simulink model "ieee80211n"  (Simulink 6.0)
settings: Solver=VariableStepDiscrete  StartTime=0.0  StopTime=inf  RelTol=1e-3
PreLoadFcn:
  | load IEEE80211n_init;
values from neighbouring files (symbols this model uses):
  params =     [IEEE80211n_init.mat]    (also in IEEE80211n_settings.m = p)
undefined symbols (not defined in the file or in its folder): magnitude
libraries: commblkintrlv2 x196, dspsigops x143, simulink x136, commdigbbndam2 x98, dspmtrx3 x96, dspsigattribs x69, dspstat3 x38, commutil2 x32, commsequence2 x26, commcnvcod2 x10, dspindex x9, dspmlti3 x8
(part 9 of 12)

== system ieee80211n/MIMODetection/Channel Estimation/ChannelEst10 ==
  trainsig : Inport  Port=1  LatchInput=off
  rxsig : Inport  Port=2  LatchInput=off
  Channel estimates : Subsystem
  Product1 : Product  Inputs=**  SaturateOnIntegerOverflow=on
  Remove DC component : Selector  InputType=Matrix  Elements=[1:26 27:]  Rows=[1:28 30:57]  Columns=-1  InputPortWidth=53
  Remove training DC component : Selector  InputType=Matrix  Elements=[1:26 27:]  Rows=[1:28 30:57]  Columns=-1  InputPortWidth=53
  Select training/data : S-Function  AncestorBlock=dspindex/Multiport Selector  FunctionName=sdspmultiportsel  Parameters=rowsOrCols, numOutports, flatIdxVect, flatLenVect, idxErrMode  mask(Multiport Selector){rowsOrCols=Columns, idxCellArray={params.OFDM_TotPreamblePerFrame-params.OFDM_HTLTF_SymPerFrame+1:params.OFDM_TotPreamblePerFrame}, idxErrMode=Clip Index}
      mask prompts: rowsOrCols "Select:"; idxCellArray "Indices to output:"; idxErrMode "Invalid index:"
      mask help: Output specified rows or columns to one or more output ports. The number of output ports is determined by the number of index vectors, each specified as a separate vector entry in a cell array. Indices are 1-based and need not be unique.
      mask init:
      | [numOutports, flatLenVect, flatIdxVect] = dspblkmultiportsel(idxCellArray);
      mask Help: web(dspbhelp);
      mask StyleString: popup(Rows|Columns),edit,popup(Clip Index|Clip and Warn|Generate Error)
      mask Display: disp(['Select\n' &1]);
  out : Outport
  wires:
  rxsig/1 -> Remove DC component/1
  Channel estimates/1(ch est) -> out/1
  trainsig/1 -> Remove training DC component/1
  Product1/1 -> Channel estimates/2(in)
  Select training/data/1 -> Product1/2
  Remove DC component/1 -> Select training/data/1
  Remove training DC component/1 -> Product1/1, Channel estimates/1(trn)

== system ieee80211n/MIMODetection/Channel Estimation/ChannelEst11 ==
  trainsig : Inport  Port=1  LatchInput=off
  rxsig : Inport  Port=2  LatchInput=off
  Channel estimates : Subsystem
  Product1 : Product  Inputs=**  SaturateOnIntegerOverflow=on
  Remove DC component : Selector  InputType=Matrix  Elements=[1:26 27:]  Rows=[1:28 30:57]  Columns=-1  InputPortWidth=53
  Remove training DC component : Selector  InputType=Matrix  Elements=[1:26 27:]  Rows=[1:28 30:57]  Columns=-1  InputPortWidth=53
  Select training/data : S-Function  AncestorBlock=dspindex/Multiport Selector  FunctionName=sdspmultiportsel  Parameters=rowsOrCols, numOutports, flatIdxVect, flatLenVect, idxErrMode  mask(Multiport Selector){rowsOrCols=Columns, idxCellArray={params.OFDM_TotPreamblePerFrame-params.OFDM_HTLTF_SymPerFrame+1:params.OFDM_TotPreamblePerFrame}, idxErrMode=Clip Index}
      mask prompts: rowsOrCols "Select:"; idxCellArray "Indices to output:"; idxErrMode "Invalid index:"
      mask help: Output specified rows or columns to one or more output ports. The number of output ports is determined by the number of index vectors, each specified as a separate vector entry in a cell array. Indices are 1-based and need not be unique.
      mask init:
      | [numOutports, flatLenVect, flatIdxVect] = dspblkmultiportsel(idxCellArray);
      mask Help: web(dspbhelp);
      mask StyleString: popup(Rows|Columns),edit,popup(Clip Index|Clip and Warn|Generate Error)
      mask Display: disp(['Select\n' &1]);
  out : Outport
  wires:
  rxsig/1 -> Remove DC component/1
  Channel estimates/1(ch est) -> out/1
  trainsig/1 -> Remove training DC component/1
  Product1/1 -> Channel estimates/2(in)
  Select training/data/1 -> Product1/2
  Remove DC component/1 -> Select training/data/1
  Remove training DC component/1 -> Product1/1, Channel estimates/1(trn)

== system ieee80211n/MIMODetection/Channel Estimation/ChannelEst12 ==
  trainsig : Inport  Port=1  LatchInput=off
  rxsig : Inport  Port=2  LatchInput=off
  Channel estimates : Subsystem
  Product1 : Product  Inputs=**  SaturateOnIntegerOverflow=on
  Remove DC component : Selector  InputType=Matrix  Elements=[1:26 27:]  Rows=[1:28 30:57]  Columns=-1  InputPortWidth=53
  Remove training DC component : Selector  InputType=Matrix  Elements=[1:26 27:]  Rows=[1:28 30:57]  Columns=-1  InputPortWidth=53
  Select training/data : S-Function  AncestorBlock=dspindex/Multiport Selector  FunctionName=sdspmultiportsel  Parameters=rowsOrCols, numOutports, flatIdxVect, flatLenVect, idxErrMode  mask(Multiport Selector){rowsOrCols=Columns, idxCellArray={params.OFDM_TotPreamblePerFrame-params.OFDM_HTLTF_SymPerFrame+1:params.OFDM_TotPreamblePerFrame}, idxErrMode=Clip Index}
      mask prompts: rowsOrCols "Select:"; idxCellArray "Indices to output:"; idxErrMode "Invalid index:"
      mask help: Output specified rows or columns to one or more output ports. The number of output ports is determined by the number of index vectors, each specified as a separate vector entry in a cell array. Indices are 1-based and need not be unique.
      mask init:
      | [numOutports, flatLenVect, flatIdxVect] = dspblkmultiportsel(idxCellArray);
      mask Help: web(dspbhelp);
      mask StyleString: popup(Rows|Columns),edit,popup(Clip Index|Clip and Warn|Generate Error)
      mask Display: disp(['Select\n' &1]);
  out : Outport
  wires:
  rxsig/1 -> Remove DC component/1
  Channel estimates/1(ch est) -> out/1
  trainsig/1 -> Remove training DC component/1
  Product1/1 -> Channel estimates/2(in)
  Select training/data/1 -> Product1/2
  Remove DC component/1 -> Select training/data/1
  Remove training DC component/1 -> Product1/1, Channel estimates/1(trn)

== system ieee80211n/MIMODetection/Channel Estimation/ChannelEst13 ==
  trainsig : Inport  Port=1  LatchInput=off
  rxsig : Inport  Port=2  LatchInput=off
  Channel estimates : Subsystem
  Product1 : Product  Inputs=**  SaturateOnIntegerOverflow=on
  Remove DC component : Selector  InputType=Matrix  Elements=[1:26 27:]  Rows=[1:28 30:57]  Columns=-1  InputPortWidth=53
  Remove training DC component : Selector  InputType=Matrix  Elements=[1:26 27:]  Rows=[1:28 30:57]  Columns=-1  InputPortWidth=53
  Select training/data : S-Function  AncestorBlock=dspindex/Multiport Selector  FunctionName=sdspmultiportsel  Parameters=rowsOrCols, numOutports, flatIdxVect, flatLenVect, idxErrMode  mask(Multiport Selector){rowsOrCols=Columns, idxCellArray={params.OFDM_TotPreamblePerFrame-params.OFDM_HTLTF_SymPerFrame+1:params.OFDM_TotPreamblePerFrame}, idxErrMode=Clip Index}
      mask prompts: rowsOrCols "Select:"; idxCellArray "Indices to output:"; idxErrMode "Invalid index:"
      mask help: Output specified rows or columns to one or more output ports. The number of output ports is determined by the number of index vectors, each specified as a separate vector entry in a cell array. Indices are 1-based and need not be unique.
      mask init:
      | [numOutports, flatLenVect, flatIdxVect] = dspblkmultiportsel(idxCellArray);
      mask Help: web(dspbhelp);
      mask StyleString: popup(Rows|Columns),edit,popup(Clip Index|Clip and Warn|Generate Error)
      mask Display: disp(['Select\n' &1]);
  out : Outport
  wires:
  rxsig/1 -> Remove DC component/1
  Channel estimates/1(ch est) -> out/1
  trainsig/1 -> Remove training DC component/1
  Product1/1 -> Channel estimates/2(in)
  Select training/data/1 -> Product1/2
  Remove DC component/1 -> Select training/data/1
  Remove training DC component/1 -> Product1/1, Channel estimates/1(trn)

== system ieee80211n/MIMODetection/Channel Estimation/ChannelEst14 ==
  trainsig : Inport  Port=1  LatchInput=off
  rxsig : Inport  Port=2  LatchInput=off
  Channel estimates : Subsystem
  Product1 : Product  Inputs=**  SaturateOnIntegerOverflow=on
  Remove DC component : Selector  InputType=Matrix  Elements=[1:26 27:]  Rows=[1:28 30:57]  Columns=-1  InputPortWidth=53
  Remove training DC component : Selector  InputType=Matrix  Elements=[1:26 27:]  Rows=[1:28 30:57]  Columns=-1  InputPortWidth=53
  Select training/data : S-Function  AncestorBlock=dspindex/Multiport Selector  FunctionName=sdspmultiportsel  Parameters=rowsOrCols, numOutports, flatIdxVect, flatLenVect, idxErrMode  mask(Multiport Selector){rowsOrCols=Columns, idxCellArray={params.OFDM_TotPreamblePerFrame-params.OFDM_HTLTF_SymPerFrame+1:params.OFDM_TotPreamblePerFrame}, idxErrMode=Clip Index}
      mask prompts: rowsOrCols "Select:"; idxCellArray "Indices to output:"; idxErrMode "Invalid index:"
      mask help: Output specified rows or columns to one or more output ports. The number of output ports is determined by the number of index vectors, each specified as a separate vector entry in a cell array. Indices are 1-based and need not be unique.
      mask init:
      | [numOutports, flatLenVect, flatIdxVect] = dspblkmultiportsel(idxCellArray);
      mask Help: web(dspbhelp);
      mask StyleString: popup(Rows|Columns),edit,popup(Clip Index|Clip and Warn|Generate Error)
      mask Display: disp(['Select\n' &1]);
  out : Outport
  wires:
  rxsig/1 -> Remove DC component/1
  Channel estimates/1(ch est) -> out/1
  trainsig/1 -> Remove training DC component/1
  Product1/1 -> Channel estimates/2(in)
  Select training/data/1 -> Product1/2
  Remove DC component/1 -> Select training/data/1
  Remove training DC component/1 -> Product1/1, Channel estimates/1(trn)

== system ieee80211n/MIMODetection/Channel Estimation/ChannelEst15 ==
  trainsig : Inport  Port=1  LatchInput=off
  rxsig : Inport  Port=2  LatchInput=off
  Channel estimates : Subsystem
  Product1 : Product  Inputs=**  SaturateOnIntegerOverflow=on
  Remove DC component : Selector  InputType=Matrix  Elements=[1:26 27:]  Rows=[1:28 30:57]  Columns=-1  InputPortWidth=53
  Remove training DC component : Selector  InputType=Matrix  Elements=[1:26 27:]  Rows=[1:28 30:57]  Columns=-1  InputPortWidth=53
  Select training/data : S-Function  AncestorBlock=dspindex/Multiport Selector  FunctionName=sdspmultiportsel  Parameters=rowsOrCols, numOutports, flatIdxVect, flatLenVect, idxErrMode  mask(Multiport Selector){rowsOrCols=Columns, idxCellArray={params.OFDM_TotPreamblePerFrame-params.OFDM_HTLTF_SymPerFrame+1:params.OFDM_TotPreamblePerFrame}, idxErrMode=Clip Index}
      mask prompts: rowsOrCols "Select:"; idxCellArray "Indices to output:"; idxErrMode "Invalid index:"
      mask help: Output specified rows or columns to one or more output ports. The number of output ports is determined by the number of index vectors, each specified as a separate vector entry in a cell array. Indices are 1-based and need not be unique.
      mask init:
      | [numOutports, flatLenVect, flatIdxVect] = dspblkmultiportsel(idxCellArray);
      mask Help: web(dspbhelp);
      mask StyleString: popup(Rows|Columns),edit,popup(Clip Index|Clip and Warn|Generate Error)
      mask Display: disp(['Select\n' &1]);
  out : Outport
  wires:
  rxsig/1 -> Remove DC component/1
  Channel estimates/1(ch est) -> out/1
  trainsig/1 -> Remove training DC component/1
  Product1/1 -> Channel estimates/2(in)
  Select training/data/1 -> Product1/2
  Remove DC component/1 -> Select training/data/1
  Remove training DC component/1 -> Product1/1, Channel estimates/1(trn)

== system ieee80211n/MIMODetection/Channel Estimation/ChannelEst16 ==
  trainsig : Inport  Port=1  LatchInput=off
  rxsig : Inport  Port=2  LatchInput=off
  Channel estimates : Subsystem
  Product1 : Product  Inputs=**  SaturateOnIntegerOverflow=on
  Remove DC component : Selector  InputType=Matrix  Elements=[1:26 27:]  Rows=[1:28 30:57]  Columns=-1  InputPortWidth=53
  Remove training DC component : Selector  InputType=Matrix  Elements=[1:26 27:]  Rows=[1:28 30:57]  Columns=-1  InputPortWidth=53
  Select training/data : S-Function  AncestorBlock=dspindex/Multiport Selector  FunctionName=sdspmultiportsel  Parameters=rowsOrCols, numOutports, flatIdxVect, flatLenVect, idxErrMode  mask(Multiport Selector){rowsOrCols=Columns, idxCellArray={params.OFDM_TotPreamblePerFrame-params.OFDM_HTLTF_SymPerFrame+1:params.OFDM_TotPreamblePerFrame}, idxErrMode=Clip Index}
      mask prompts: rowsOrCols "Select:"; idxCellArray "Indices to output:"; idxErrMode "Invalid index:"
      mask help: Output specified rows or columns to one or more output ports. The number of output ports is determined by the number of index vectors, each specified as a separate vector entry in a cell array. Indices are 1-based and need not be unique.
      mask init:
      | [numOutports, flatLenVect, flatIdxVect] = dspblkmultiportsel(idxCellArray);
      mask Help: web(dspbhelp);
      mask StyleString: popup(Rows|Columns),edit,popup(Clip Index|Clip and Warn|Generate Error)
      mask Display: disp(['Select\n' &1]);
  out : Outport
  wires:
  rxsig/1 -> Remove DC component/1
  Channel estimates/1(ch est) -> out/1
  trainsig/1 -> Remove training DC component/1
  Product1/1 -> Channel estimates/2(in)
  Select training/data/1 -> Product1/2
  Remove DC component/1 -> Select training/data/1
  Remove training DC component/1 -> Product1/1, Channel estimates/1(trn)

== system ieee80211n/MIMODetection/Channel Estimation/ChannelEst2 ==
  trainsig : Inport  Port=1  LatchInput=off
  rxsig : Inport  Port=2  LatchInput=off
  Channel estimates : Subsystem
  Product1 : Product  Inputs=**  SaturateOnIntegerOverflow=on
  Remove DC component : Selector  InputType=Matrix  Elements=[1:26 27:]  Rows=[1:28 30:57]  Columns=-1  InputPortWidth=53
  Remove training DC component : Selector  InputType=Matrix  Elements=[1:26 27:]  Rows=[1:28 30:57]  Columns=-1  InputPortWidth=53
  Select training/data : S-Function  AncestorBlock=dspindex/Multiport Selector  FunctionName=sdspmultiportsel  Parameters=rowsOrCols, numOutports, flatIdxVect, flatLenVect, idxErrMode  mask(Multiport Selector){rowsOrCols=Columns, idxCellArray={params.OFDM_TotPreamblePerFrame-params.OFDM_HTLTF_SymPerFrame+1:params.OFDM_TotPreamblePerFrame}, idxErrMode=Clip Index}
      mask prompts: rowsOrCols "Select:"; idxCellArray "Indices to output:"; idxErrMode "Invalid index:"
      mask help: Output specified rows or columns to one or more output ports. The number of output ports is determined by the number of index vectors, each specified as a separate vector entry in a cell array. Indices are 1-based and need not be unique.
      mask init:
      | [numOutports, flatLenVect, flatIdxVect] = dspblkmultiportsel(idxCellArray);
      mask Help: web(dspbhelp);
      mask StyleString: popup(Rows|Columns),edit,popup(Clip Index|Clip and Warn|Generate Error)
      mask Display: disp(['Select\n' &1]);
  out : Outport
  wires:
  rxsig/1 -> Remove DC component/1
  Channel estimates/1(ch est) -> out/1
  trainsig/1 -> Remove training DC component/1
  Product1/1 -> Channel estimates/2(in)
  Select training/data/1 -> Product1/2
  Remove DC component/1 -> Select training/data/1
  Remove training DC component/1 -> Product1/1, Channel estimates/1(trn)

== system ieee80211n/MIMODetection/Channel Estimation/ChannelEst3 ==
  trainsig : Inport  Port=1  LatchInput=off
  rxsig : Inport  Port=2  LatchInput=off
  Channel estimates : Subsystem
  Product1 : Product  Inputs=**  SaturateOnIntegerOverflow=on
  Remove DC component : Selector  InputType=Matrix  Elements=[1:26 27:]  Rows=[1:28 30:57]  Columns=-1  InputPortWidth=53
  Remove training DC component : Selector  InputType=Matrix  Elements=[1:26 27:]  Rows=[1:28 30:57]  Columns=-1  InputPortWidth=53
  Select training/data : S-Function  AncestorBlock=dspindex/Multiport Selector  FunctionName=sdspmultiportsel  Parameters=rowsOrCols, numOutports, flatIdxVect, flatLenVect, idxErrMode  mask(Multiport Selector){rowsOrCols=Columns, idxCellArray={params.OFDM_TotPreamblePerFrame-params.OFDM_HTLTF_SymPerFrame+1:params.OFDM_TotPreamblePerFrame}, idxErrMode=Clip Index}
      mask prompts: rowsOrCols "Select:"; idxCellArray "Indices to output:"; idxErrMode "Invalid index:"
      mask help: Output specified rows or columns to one or more output ports. The number of output ports is determined by the number of index vectors, each specified as a separate vector entry in a cell array. Indices are 1-based and need not be unique.
      mask init:
      | [numOutports, flatLenVect, flatIdxVect] = dspblkmultiportsel(idxCellArray);
      mask Help: web(dspbhelp);
      mask StyleString: popup(Rows|Columns),edit,popup(Clip Index|Clip and Warn|Generate Error)
      mask Display: disp(['Select\n' &1]);
  out : Outport
  wires:
  rxsig/1 -> Remove DC component/1
  Channel estimates/1(ch est) -> out/1
  trainsig/1 -> Remove training DC component/1
  Product1/1 -> Channel estimates/2(in)
  Select training/data/1 -> Product1/2
  Remove DC component/1 -> Select training/data/1
  Remove training DC component/1 -> Product1/1, Channel estimates/1(trn)

== system ieee80211n/MIMODetection/Channel Estimation/ChannelEst4 ==
  trainsig : Inport  Port=1  LatchInput=off
  rxsig : Inport  Port=2  LatchInput=off
  Channel estimates : Subsystem
  Product1 : Product  Inputs=**  SaturateOnIntegerOverflow=on
  Remove DC component : Selector  InputType=Matrix  Elements=[1:26 27:]  Rows=[1:28 30:57]  Columns=-1  InputPortWidth=53
  Remove training DC component : Selector  InputType=Matrix  Elements=[1:26 27:]  Rows=[1:28 30:57]  Columns=-1  InputPortWidth=53
  Select training/data : S-Function  AncestorBlock=dspindex/Multiport Selector  FunctionName=sdspmultiportsel  Parameters=rowsOrCols, numOutports, flatIdxVect, flatLenVect, idxErrMode  mask(Multiport Selector){rowsOrCols=Columns, idxCellArray={params.OFDM_TotPreamblePerFrame-params.OFDM_HTLTF_SymPerFrame+1:params.OFDM_TotPreamblePerFrame}, idxErrMode=Clip Index}
      mask prompts: rowsOrCols "Select:"; idxCellArray "Indices to output:"; idxErrMode "Invalid index:"
      mask help: Output specified rows or columns to one or more output ports. The number of output ports is determined by the number of index vectors, each specified as a separate vector entry in a cell array. Indices are 1-based and need not be unique.
      mask init:
      | [numOutports, flatLenVect, flatIdxVect] = dspblkmultiportsel(idxCellArray);
      mask Help: web(dspbhelp);
      mask StyleString: popup(Rows|Columns),edit,popup(Clip Index|Clip and Warn|Generate Error)
      mask Display: disp(['Select\n' &1]);
  out : Outport
  wires:
  rxsig/1 -> Remove DC component/1
  Channel estimates/1(ch est) -> out/1
  trainsig/1 -> Remove training DC component/1
  Product1/1 -> Channel estimates/2(in)
  Select training/data/1 -> Product1/2
  Remove DC component/1 -> Select training/data/1
  Remove training DC component/1 -> Product1/1, Channel estimates/1(trn)

== system ieee80211n/MIMODetection/Channel Estimation/ChannelEst5 ==
  trainsig : Inport  Port=1  LatchInput=off
  rxsig : Inport  Port=2  LatchInput=off
  Channel estimates : Subsystem
  Product1 : Product  Inputs=**  SaturateOnIntegerOverflow=on
  Remove DC component : Selector  InputType=Matrix  Elements=[1:26 27:]  Rows=[1:28 30:57]  Columns=-1  InputPortWidth=53
  Remove training DC component : Selector  InputType=Matrix  Elements=[1:26 27:]  Rows=[1:28 30:57]  Columns=-1  InputPortWidth=53
  Select training/data : S-Function  AncestorBlock=dspindex/Multiport Selector  FunctionName=sdspmultiportsel  Parameters=rowsOrCols, numOutports, flatIdxVect, flatLenVect, idxErrMode  mask(Multiport Selector){rowsOrCols=Columns, idxCellArray={params.OFDM_TotPreamblePerFrame-params.OFDM_HTLTF_SymPerFrame+1:params.OFDM_TotPreamblePerFrame}, idxErrMode=Clip Index}
      mask prompts: rowsOrCols "Select:"; idxCellArray "Indices to output:"; idxErrMode "Invalid index:"
      mask help: Output specified rows or columns to one or more output ports. The number of output ports is determined by the number of index vectors, each specified as a separate vector entry in a cell array. Indices are 1-based and need not be unique.
      mask init:
      | [numOutports, flatLenVect, flatIdxVect] = dspblkmultiportsel(idxCellArray);
      mask Help: web(dspbhelp);
      mask StyleString: popup(Rows|Columns),edit,popup(Clip Index|Clip and Warn|Generate Error)
      mask Display: disp(['Select\n' &1]);
  out : Outport
  wires:
  rxsig/1 -> Remove DC component/1
  Channel estimates/1(ch est) -> out/1
  trainsig/1 -> Remove training DC component/1
  Product1/1 -> Channel estimates/2(in)
  Select training/data/1 -> Product1/2
  Remove DC component/1 -> Select training/data/1
  Remove training DC component/1 -> Product1/1, Channel estimates/1(trn)

== system ieee80211n/MIMODetection/Channel Estimation/ChannelEst6 ==
  trainsig : Inport  Port=1  LatchInput=off
  rxsig : Inport  Port=2  LatchInput=off
  Channel estimates : Subsystem
  Product1 : Product  Inputs=**  SaturateOnIntegerOverflow=on
  Remove DC component : Selector  InputType=Matrix  Elements=[1:26 27:]  Rows=[1:28 30:57]  Columns=-1  InputPortWidth=53
  Remove training DC component : Selector  InputType=Matrix  Elements=[1:26 27:]  Rows=[1:28 30:57]  Columns=-1  InputPortWidth=53
  Select training/data : S-Function  AncestorBlock=dspindex/Multiport Selector  FunctionName=sdspmultiportsel  Parameters=rowsOrCols, numOutports, flatIdxVect, flatLenVect, idxErrMode  mask(Multiport Selector){rowsOrCols=Columns, idxCellArray={params.OFDM_TotPreamblePerFrame-params.OFDM_HTLTF_SymPerFrame+1:params.OFDM_TotPreamblePerFrame}, idxErrMode=Clip Index}
      mask prompts: rowsOrCols "Select:"; idxCellArray "Indices to output:"; idxErrMode "Invalid index:"
      mask help: Output specified rows or columns to one or more output ports. The number of output ports is determined by the number of index vectors, each specified as a separate vector entry in a cell array. Indices are 1-based and need not be unique.
      mask init:
      | [numOutports, flatLenVect, flatIdxVect] = dspblkmultiportsel(idxCellArray);
      mask Help: web(dspbhelp);
      mask StyleString: popup(Rows|Columns),edit,popup(Clip Index|Clip and Warn|Generate Error)
      mask Display: disp(['Select\n' &1]);
  out : Outport
  wires:
  rxsig/1 -> Remove DC component/1
  Channel estimates/1(ch est) -> out/1
  trainsig/1 -> Remove training DC component/1
  Product1/1 -> Channel estimates/2(in)
  Select training/data/1 -> Product1/2
  Remove DC component/1 -> Select training/data/1
  Remove training DC component/1 -> Product1/1, Channel estimates/1(trn)

== system ieee80211n/MIMODetection/Channel Estimation/ChannelEst7 ==
  trainsig : Inport  Port=1  LatchInput=off
  rxsig : Inport  Port=2  LatchInput=off
  Channel estimates : Subsystem
  Product1 : Product  Inputs=**  SaturateOnIntegerOverflow=on
  Remove DC component : Selector  InputType=Matrix  Elements=[1:26 27:]  Rows=[1:28 30:57]  Columns=-1  InputPortWidth=53
  Remove training DC component : Selector  InputType=Matrix  Elements=[1:26 27:]  Rows=[1:28 30:57]  Columns=-1  InputPortWidth=53
  Select training/data : S-Function  AncestorBlock=dspindex/Multiport Selector  FunctionName=sdspmultiportsel  Parameters=rowsOrCols, numOutports, flatIdxVect, flatLenVect, idxErrMode  mask(Multiport Selector){rowsOrCols=Columns, idxCellArray={params.OFDM_TotPreamblePerFrame-params.OFDM_HTLTF_SymPerFrame+1:params.OFDM_TotPreamblePerFrame}, idxErrMode=Clip Index}
      mask prompts: rowsOrCols "Select:"; idxCellArray "Indices to output:"; idxErrMode "Invalid index:"
      mask help: Output specified rows or columns to one or more output ports. The number of output ports is determined by the number of index vectors, each specified as a separate vector entry in a cell array. Indices are 1-based and need not be unique.
      mask init:
      | [numOutports, flatLenVect, flatIdxVect] = dspblkmultiportsel(idxCellArray);
      mask Help: web(dspbhelp);
      mask StyleString: popup(Rows|Columns),edit,popup(Clip Index|Clip and Warn|Generate Error)
      mask Display: disp(['Select\n' &1]);
  out : Outport
  wires:
  rxsig/1 -> Remove DC component/1
  Channel estimates/1(ch est) -> out/1
  trainsig/1 -> Remove training DC component/1
  Product1/1 -> Channel estimates/2(in)
  Select training/data/1 -> Product1/2
  Remove DC component/1 -> Select training/data/1
  Remove training DC component/1 -> Product1/1, Channel estimates/1(trn)

== system ieee80211n/MIMODetection/Channel Estimation/ChannelEst8 ==
  trainsig : Inport  Port=1  LatchInput=off
  rxsig : Inport  Port=2  LatchInput=off
  Channel estimates : Subsystem
  Product1 : Product  Inputs=**  SaturateOnIntegerOverflow=on
  Remove DC component : Selector  InputType=Matrix  Elements=[1:26 27:]  Rows=[1:28 30:57]  Columns=-1  InputPortWidth=53
  Remove training DC component : Selector  InputType=Matrix  Elements=[1:26 27:]  Rows=[1:28 30:57]  Columns=-1  InputPortWidth=53
  Select training/data : S-Function  AncestorBlock=dspindex/Multiport Selector  FunctionName=sdspmultiportsel  Parameters=rowsOrCols, numOutports, flatIdxVect, flatLenVect, idxErrMode  mask(Multiport Selector){rowsOrCols=Columns, idxCellArray={params.OFDM_TotPreamblePerFrame-params.OFDM_HTLTF_SymPerFrame+1:params.OFDM_TotPreamblePerFrame}, idxErrMode=Clip Index}
      mask prompts: rowsOrCols "Select:"; idxCellArray "Indices to output:"; idxErrMode "Invalid index:"
      mask help: Output specified rows or columns to one or more output ports. The number of output ports is determined by the number of index vectors, each specified as a separate vector entry in a cell array. Indices are 1-based and need not be unique.
      mask init:
      | [numOutports, flatLenVect, flatIdxVect] = dspblkmultiportsel(idxCellArray);
      mask Help: web(dspbhelp);
      mask StyleString: popup(Rows|Columns),edit,popup(Clip Index|Clip and Warn|Generate Error)
      mask Display: disp(['Select\n' &1]);
  out : Outport
  wires:
  rxsig/1 -> Remove DC component/1
  Channel estimates/1(ch est) -> out/1
  trainsig/1 -> Remove training DC component/1
  Product1/1 -> Channel estimates/2(in)
  Select training/data/1 -> Product1/2
  Remove DC component/1 -> Select training/data/1
  Remove training DC component/1 -> Product1/1, Channel estimates/1(trn)

== system ieee80211n/MIMODetection/Channel Estimation/ChannelEst9 ==
  trainsig : Inport  Port=1  LatchInput=off
  rxsig : Inport  Port=2  LatchInput=off
  Channel estimates : Subsystem
  Product1 : Product  Inputs=**  SaturateOnIntegerOverflow=on
  Remove DC component : Selector  InputType=Matrix  Elements=[1:26 27:]  Rows=[1:28 30:57]  Columns=-1  InputPortWidth=53
  Remove training DC component : Selector  InputType=Matrix  Elements=[1:26 27:]  Rows=[1:28 30:57]  Columns=-1  InputPortWidth=53
  Select training/data : S-Function  AncestorBlock=dspindex/Multiport Selector  FunctionName=sdspmultiportsel  Parameters=rowsOrCols, numOutports, flatIdxVect, flatLenVect, idxErrMode  mask(Multiport Selector){rowsOrCols=Columns, idxCellArray={params.OFDM_TotPreamblePerFrame-params.OFDM_HTLTF_SymPerFrame+1:params.OFDM_TotPreamblePerFrame}, idxErrMode=Clip Index}
      mask prompts: rowsOrCols "Select:"; idxCellArray "Indices to output:"; idxErrMode "Invalid index:"
      mask help: Output specified rows or columns to one or more output ports. The number of output ports is determined by the number of index vectors, each specified as a separate vector entry in a cell array. Indices are 1-based and need not be unique.
      mask init:
      | [numOutports, flatLenVect, flatIdxVect] = dspblkmultiportsel(idxCellArray);
      mask Help: web(dspbhelp);
      mask StyleString: popup(Rows|Columns),edit,popup(Clip Index|Clip and Warn|Generate Error)
      mask Display: disp(['Select\n' &1]);
  out : Outport
  wires:
  rxsig/1 -> Remove DC component/1
  Channel estimates/1(ch est) -> out/1
  trainsig/1 -> Remove training DC component/1
  Product1/1 -> Channel estimates/2(in)
  Select training/data/1 -> Product1/2
  Remove DC component/1 -> Select training/data/1
  Remove training DC component/1 -> Product1/1, Channel estimates/1(trn)

== system ieee80211n/ModulatorBank/CC_PuncBank/Modulator 1 ==
  txdata : Inport  Port=1  LatchInput=off
  Enable : EnablePort
  Convolutional Encoder1 : commcnvcod2/Convolutional Encoder  trellis=trellisStructure  reset=None
  P2 Puncture : commsequence2/Puncture  punctureVector=punctureVector
  Zero Pad : dspsigops/Zero Pad  padSigAt=End  zpadAlong=Columns  padNumOutRowsSpecMethod=User-specified  numOutRows=Nb_max  padNumOutColsSpecMethod=User-specified  numOutCols=1  trunc_flag=None
      settings: AttributesFormatString=\n
  Zero Pad1 : dspsigops/Zero Pad  padSigAt=End  zpadAlong=Columns  padNumOutRowsSpecMethod=User-specified  numOutRows=bitsPerBlock  padNumOutColsSpecMethod=User-specified  numOutCols=1  trunc_flag=None
      settings: AttributesFormatString=\n
  txsig : Outport
  wires:
  txdata/1 -> Zero Pad1/1
  Convolutional Encoder1/1 -> P2 Puncture/1
  P2 Puncture/1 -> Zero Pad/1
  Zero Pad/1 -> txsig/1
  Zero Pad1/1 -> Convolutional Encoder1/1

== system ieee80211n/ModulatorBank/CC_PuncBank/Modulator 2 ==
  txdata : Inport  Port=1  LatchInput=off
  Enable : EnablePort
  Convolutional Encoder1 : commcnvcod2/Convolutional Encoder  trellis=trellisStructure  reset=None
  P2 Puncture : commsequence2/Puncture  punctureVector=punctureVector
  Zero Pad : dspsigops/Zero Pad  padSigAt=End  zpadAlong=Columns  padNumOutRowsSpecMethod=User-specified  numOutRows=Nb_max  padNumOutColsSpecMethod=User-specified  numOutCols=1  trunc_flag=None
      settings: AttributesFormatString=\n
  Zero Pad1 : dspsigops/Zero Pad  padSigAt=End  zpadAlong=Columns  padNumOutRowsSpecMethod=User-specified  numOutRows=bitsPerBlock  padNumOutColsSpecMethod=User-specified  numOutCols=1  trunc_flag=None
      settings: AttributesFormatString=\n
  txsig : Outport
  wires:
  txdata/1 -> Zero Pad1/1
  Convolutional Encoder1/1 -> P2 Puncture/1
  P2 Puncture/1 -> Zero Pad/1
  Zero Pad/1 -> txsig/1
  Zero Pad1/1 -> Convolutional Encoder1/1

== system ieee80211n/ModulatorBank/CC_PuncBank/Modulator 3 ==
  txdata : Inport  Port=1  LatchInput=off
  Enable : EnablePort
  Convolutional Encoder1 : commcnvcod2/Convolutional Encoder  trellis=trellisStructure  reset=None
  P2 Puncture : commsequence2/Puncture  punctureVector=punctureVector
  Zero Pad : dspsigops/Zero Pad  padSigAt=End  zpadAlong=Columns  padNumOutRowsSpecMethod=User-specified  numOutRows=Nb_max  padNumOutColsSpecMethod=User-specified  numOutCols=1  trunc_flag=None
      settings: AttributesFormatString=\n
  Zero Pad1 : dspsigops/Zero Pad  padSigAt=End  zpadAlong=Columns  padNumOutRowsSpecMethod=User-specified  numOutRows=bitsPerBlock  padNumOutColsSpecMethod=User-specified  numOutCols=1  trunc_flag=None
      settings: AttributesFormatString=\n
  txsig : Outport
  wires:
  txdata/1 -> Zero Pad1/1
  Convolutional Encoder1/1 -> P2 Puncture/1
  P2 Puncture/1 -> Zero Pad/1
  Zero Pad/1 -> txsig/1
  Zero Pad1/1 -> Convolutional Encoder1/1

== system ieee80211n/ModulatorBank/CC_PuncBank/Modulator 4 ==
  txdata : Inport  Port=1  LatchInput=off
  Enable : EnablePort
  Convolutional Encoder1 : commcnvcod2/Convolutional Encoder  trellis=trellisStructure  reset=None
  P2 Puncture : commsequence2/Puncture  punctureVector=punctureVector
  Zero Pad : dspsigops/Zero Pad  padSigAt=End  zpadAlong=Columns  padNumOutRowsSpecMethod=User-specified  numOutRows=Nb_max  padNumOutColsSpecMethod=User-specified  numOutCols=1  trunc_flag=None
      settings: AttributesFormatString=\n
  Zero Pad1 : dspsigops/Zero Pad  padSigAt=End  zpadAlong=Columns  padNumOutRowsSpecMethod=User-specified  numOutRows=bitsPerBlock  padNumOutColsSpecMethod=User-specified  numOutCols=1  trunc_flag=None
      settings: AttributesFormatString=\n
  txsig : Outport
  wires:
  txdata/1 -> Zero Pad1/1
  Convolutional Encoder1/1 -> P2 Puncture/1
  P2 Puncture/1 -> Zero Pad/1
  Zero Pad/1 -> txsig/1
  Zero Pad1/1 -> Convolutional Encoder1/1

== system ieee80211n/ModulatorBank/CC_PuncBank/Modulator 5 ==
  txdata : Inport  Port=1  LatchInput=off
  Enable : EnablePort
  Convolutional Encoder1 : commcnvcod2/Convolutional Encoder  trellis=trellisStructure  reset=None
  P2 Puncture : commsequence2/Puncture  punctureVector=punctureVector
  Zero Pad : dspsigops/Zero Pad  padSigAt=End  zpadAlong=Columns  padNumOutRowsSpecMethod=User-specified  numOutRows=Nb_max  padNumOutColsSpecMethod=User-specified  numOutCols=1  trunc_flag=None
      settings: AttributesFormatString=\n
  Zero Pad1 : dspsigops/Zero Pad  padSigAt=End  zpadAlong=Columns  padNumOutRowsSpecMethod=User-specified  numOutRows=bitsPerBlock  padNumOutColsSpecMethod=User-specified  numOutCols=1  trunc_flag=None
      settings: AttributesFormatString=\n
  txsig : Outport
  wires:
  txdata/1 -> Zero Pad1/1
  Convolutional Encoder1/1 -> P2 Puncture/1
  P2 Puncture/1 -> Zero Pad/1
  Zero Pad/1 -> txsig/1
  Zero Pad1/1 -> Convolutional Encoder1/1

== system ieee80211n/ModulatorBank/CC_PuncBank/Modulator 6 ==
  txdata : Inport  Port=1  LatchInput=off
  Enable : EnablePort
  Convolutional Encoder1 : commcnvcod2/Convolutional Encoder  trellis=trellisStructure  reset=None
  P2 Puncture : commsequence2/Puncture  punctureVector=punctureVector
  Zero Pad : dspsigops/Zero Pad  padSigAt=End  zpadAlong=Columns  padNumOutRowsSpecMethod=User-specified  numOutRows=Nb_max  padNumOutColsSpecMethod=User-specified  numOutCols=1  trunc_flag=None
      settings: AttributesFormatString=\n
  Zero Pad1 : dspsigops/Zero Pad  padSigAt=End  zpadAlong=Columns  padNumOutRowsSpecMethod=User-specified  numOutRows=bitsPerBlock  padNumOutColsSpecMethod=User-specified  numOutCols=1  trunc_flag=None
      settings: AttributesFormatString=\n
  txsig : Outport
  wires:
  txdata/1 -> Zero Pad1/1
  Convolutional Encoder1/1 -> P2 Puncture/1
  P2 Puncture/1 -> Zero Pad/1
  Zero Pad/1 -> txsig/1
  Zero Pad1/1 -> Convolutional Encoder1/1

== system ieee80211n/ModulatorBank/CC_PuncBank/Modulator 7 ==
  txdata : Inport  Port=1  LatchInput=off
  Enable : EnablePort
  Convolutional Encoder1 : commcnvcod2/Convolutional Encoder  trellis=trellisStructure  reset=None
  P2 Puncture : commsequence2/Puncture  punctureVector=punctureVector
  Zero Pad : dspsigops/Zero Pad  padSigAt=End  zpadAlong=Columns  padNumOutRowsSpecMethod=User-specified  numOutRows=Nb_max  padNumOutColsSpecMethod=User-specified  numOutCols=1  trunc_flag=None
      settings: AttributesFormatString=\n
  Zero Pad1 : dspsigops/Zero Pad  padSigAt=End  zpadAlong=Columns  padNumOutRowsSpecMethod=User-specified  numOutRows=bitsPerBlock  padNumOutColsSpecMethod=User-specified  numOutCols=1  trunc_flag=None
      settings: AttributesFormatString=\n
  txsig : Outport
  wires:
  txdata/1 -> Zero Pad1/1
  Convolutional Encoder1/1 -> P2 Puncture/1
  P2 Puncture/1 -> Zero Pad/1
  Zero Pad/1 -> txsig/1
  Zero Pad1/1 -> Convolutional Encoder1/1

== system ieee80211n/ModulatorBank/CC_PuncBank/Modulator 8 ==
  txdata : Inport  Port=1  LatchInput=off
  Enable : EnablePort
  Convolutional Encoder1 : commcnvcod2/Convolutional Encoder  trellis=trellisStructure  reset=None
  P2 Puncture : commsequence2/Puncture  punctureVector=punctureVector
  Zero Pad : dspsigops/Zero Pad  padSigAt=End  zpadAlong=Columns  padNumOutRowsSpecMethod=User-specified  numOutRows=Nb_max  padNumOutColsSpecMethod=User-specified  numOutCols=1  trunc_flag=None
      settings: AttributesFormatString=\n
  Zero Pad1 : dspsigops/Zero Pad  padSigAt=End  zpadAlong=Columns  padNumOutRowsSpecMethod=User-specified  numOutRows=bitsPerBlock  padNumOutColsSpecMethod=User-specified  numOutCols=1  trunc_flag=None
      settings: AttributesFormatString=\n
  txsig : Outport
  wires:
  txdata/1 -> Zero Pad1/1
  Convolutional Encoder1/1 -> P2 Puncture/1
  P2 Puncture/1 -> Zero Pad/1
  Zero Pad/1 -> txsig/1
  Zero Pad1/1 -> Convolutional Encoder1/1

== system ieee80211n/ModulatorBank/Group into OFDM symbols/Group into OFDM symbols ==
  in : Inport  Port=1  LatchInput=off
  Assemble Subcarriers : simulink/Math Operations/Matrix Concatenation  numInports=11  catMethod=Vertical
  DC value : Subsystem
      mask Display: disp('Zero DC')
  Pilot1 : Subsystem
      mask Display: disp('Pilot 1')
  Pilot2 : Subsystem
      mask Display: disp('Pilot 2')
  Pilot3 : Subsystem
      mask Display: disp('Pilot 3')
  Pilot4 : Subsystem
      mask Display: disp('Pilot 4')
  Select data blocks : S-Function  AncestorBlock=dspindex/Multiport Selector  FunctionName=sdspmultiportsel  Parameters=rowsOrCols, numOutports, flatIdxVect, flatLenVect, idxErrMode  mask(Multiport Selector){rowsOrCols=Rows, idxCellArray=params.TXDataCarriers, idxErrMode=Clip Index}
      mask prompts: rowsOrCols "Select:"; idxCellArray "Indices to output:"; idxErrMode "Invalid index:"
      mask help: Output specified rows or columns to one or more output ports. The number of output ports is determined by the number of index vectors, each specified as a separate vector entry in a cell array. Indices are 1-based and need not be unique.
      mask init:
      | [numOutports, flatLenVect, flatIdxVect] = dspblkmultiportsel(idxCellArray);
      mask Help: web(dspbhelp);
      mask StyleString: popup(Rows|Columns),edit,popup(Clip Index|Clip and Warn|Generate Error)
      mask Display: disp(['Select\n' &1]);
  out : Outport
  wires:
  Select data blocks/1 -> Assemble Subcarriers/1
  Select data blocks/2 -> Assemble Subcarriers/3
  Select data blocks/3 -> Assemble Subcarriers/5
  Select data blocks/4 -> Assemble Subcarriers/7
  Select data blocks/5 -> Assemble Subcarriers/9
  Select data blocks/6 -> Assemble Subcarriers/11
  Assemble Subcarriers/1 -> out/1
  DC value/1(out) -> Assemble Subcarriers/6
  in/1 -> Select data blocks/1
  Pilot1/1(out) -> Assemble Subcarriers/2
  Pilot2/1(out) -> Assemble Subcarriers/4
  Pilot3/1(out) -> Assemble Subcarriers/8
  Pilot4/1(out) -> Assemble Subcarriers/10

== system ieee80211n/ModulatorBank/Group into OFDM symbols1/Group into OFDM symbols ==
  in : Inport  Port=1  LatchInput=off
  Assemble Subcarriers : simulink/Math Operations/Matrix Concatenation  numInports=11  catMethod=Vertical
  DC value : Subsystem
      mask Display: disp('Zero DC')
  Pilot1 : Subsystem
      mask Display: disp('Pilot 1')
  Pilot2 : Subsystem
      mask Display: disp('Pilot 2')
  Pilot3 : Subsystem
      mask Display: disp('Pilot 3')
  Pilot4 : Subsystem
      mask Display: disp('Pilot 4')
  Select data blocks : S-Function  AncestorBlock=dspindex/Multiport Selector  FunctionName=sdspmultiportsel  Parameters=rowsOrCols, numOutports, flatIdxVect, flatLenVect, idxErrMode  mask(Multiport Selector){rowsOrCols=Rows, idxCellArray=params.TXDataCarriers, idxErrMode=Clip Index}
      mask prompts: rowsOrCols "Select:"; idxCellArray "Indices to output:"; idxErrMode "Invalid index:"
      mask help: Output specified rows or columns to one or more output ports. The number of output ports is determined by the number of index vectors, each specified as a separate vector entry in a cell array. Indices are 1-based and need not be unique.
      mask init:
      | [numOutports, flatLenVect, flatIdxVect] = dspblkmultiportsel(idxCellArray);
      mask Help: web(dspbhelp);
      mask StyleString: popup(Rows|Columns),edit,popup(Clip Index|Clip and Warn|Generate Error)
      mask Display: disp(['Select\n' &1]);
  out : Outport
  wires:
  Select data blocks/1 -> Assemble Subcarriers/1
  Select data blocks/2 -> Assemble Subcarriers/3
  Select data blocks/3 -> Assemble Subcarriers/5
  Select data blocks/4 -> Assemble Subcarriers/7
  Select data blocks/5 -> Assemble Subcarriers/9
  Select data blocks/6 -> Assemble Subcarriers/11
  Assemble Subcarriers/1 -> out/1
  DC value/1(out) -> Assemble Subcarriers/6
  in/1 -> Select data blocks/1
  Pilot1/1(out) -> Assemble Subcarriers/2
  Pilot2/1(out) -> Assemble Subcarriers/4
  Pilot3/1(out) -> Assemble Subcarriers/8
  Pilot4/1(out) -> Assemble Subcarriers/10

== system ieee80211n/ModulatorBank/Group into OFDM symbols2/Group into OFDM symbols ==
  in : Inport  Port=1  LatchInput=off
  Assemble Subcarriers : simulink/Math Operations/Matrix Concatenation  numInports=11  catMethod=Vertical
  DC value : Subsystem
      mask Display: disp('Zero DC')
  Pilot1 : Subsystem
      mask Display: disp('Pilot 1')
  Pilot2 : Subsystem
      mask Display: disp('Pilot 2')
  Pilot3 : Subsystem
      mask Display: disp('Pilot 3')
  Pilot4 : Subsystem
      mask Display: disp('Pilot 4')
  Select data blocks : S-Function  AncestorBlock=dspindex/Multiport Selector  FunctionName=sdspmultiportsel  Parameters=rowsOrCols, numOutports, flatIdxVect, flatLenVect, idxErrMode  mask(Multiport Selector){rowsOrCols=Rows, idxCellArray=params.TXDataCarriers, idxErrMode=Clip Index}
      mask prompts: rowsOrCols "Select:"; idxCellArray "Indices to output:"; idxErrMode "Invalid index:"
      mask help: Output specified rows or columns to one or more output ports. The number of output ports is determined by the number of index vectors, each specified as a separate vector entry in a cell array. Indices are 1-based and need not be unique.
      mask init:
      | [numOutports, flatLenVect, flatIdxVect] = dspblkmultiportsel(idxCellArray);
      mask Help: web(dspbhelp);
      mask StyleString: popup(Rows|Columns),edit,popup(Clip Index|Clip and Warn|Generate Error)
      mask Display: disp(['Select\n' &1]);
  out : Outport
  wires:
  Select data blocks/1 -> Assemble Subcarriers/1
  Select data blocks/2 -> Assemble Subcarriers/3
  Select data blocks/3 -> Assemble Subcarriers/5
  Select data blocks/4 -> Assemble Subcarriers/7
  Select data blocks/5 -> Assemble Subcarriers/9
  Select data blocks/6 -> Assemble Subcarriers/11
  Assemble Subcarriers/1 -> out/1
  DC value/1(out) -> Assemble Subcarriers/6
  in/1 -> Select data blocks/1
  Pilot1/1(out) -> Assemble Subcarriers/2
  Pilot2/1(out) -> Assemble Subcarriers/4
  Pilot3/1(out) -> Assemble Subcarriers/8
  Pilot4/1(out) -> Assemble Subcarriers/10

== system ieee80211n/ModulatorBank/Group into OFDM symbols3/Group into OFDM symbols ==
  in : Inport  Port=1  LatchInput=off
  Assemble Subcarriers : simulink/Math Operations/Matrix Concatenation  numInports=11  catMethod=Vertical
  DC value : Subsystem
      mask Display: disp('Zero DC')
  Pilot1 : Subsystem
      mask Display: disp('Pilot 1')
  Pilot2 : Subsystem
      mask Display: disp('Pilot 2')
  Pilot3 : Subsystem
      mask Display: disp('Pilot 3')
  Pilot4 : Subsystem
      mask Display: disp('Pilot 4')
  Select data blocks : S-Function  AncestorBlock=dspindex/Multiport Selector  FunctionName=sdspmultiportsel  Parameters=rowsOrCols, numOutports, flatIdxVect, flatLenVect, idxErrMode  mask(Multiport Selector){rowsOrCols=Rows, idxCellArray=params.TXDataCarriers, idxErrMode=Clip Index}
      mask prompts: rowsOrCols "Select:"; idxCellArray "Indices to output:"; idxErrMode "Invalid index:"
      mask help: Output specified rows or columns to one or more output ports. The number of output ports is determined by the number of index vectors, each specified as a separate vector entry in a cell array. Indices are 1-based and need not be unique.
      mask init:
      | [numOutports, flatLenVect, flatIdxVect] = dspblkmultiportsel(idxCellArray);
      mask Help: web(dspbhelp);
      mask StyleString: popup(Rows|Columns),edit,popup(Clip Index|Clip and Warn|Generate Error)
      mask Display: disp(['Select\n' &1]);
  out : Outport
  wires:
  Select data blocks/1 -> Assemble Subcarriers/1
  Select data blocks/2 -> Assemble Subcarriers/3
  Select data blocks/3 -> Assemble Subcarriers/5
  Select data blocks/4 -> Assemble Subcarriers/7
  Select data blocks/5 -> Assemble Subcarriers/9
  Select data blocks/6 -> Assemble Subcarriers/11
  Assemble Subcarriers/1 -> out/1
  DC value/1(out) -> Assemble Subcarriers/6
  in/1 -> Select data blocks/1
  Pilot1/1(out) -> Assemble Subcarriers/2
  Pilot2/1(out) -> Assemble Subcarriers/4
  Pilot3/1(out) -> Assemble Subcarriers/8
  Pilot4/1(out) -> Assemble Subcarriers/10

== system ieee80211n/ModulatorBank/ModulatorSS1/Modulator 1 ==
  txdata : Inport  Port=1  LatchInput=off
  Enable : EnablePort
  Gain1 : Gain  SaturateOnIntegerOverflow=on
  General Block Interleaver : commblkintrlv2/General Block Interleaver  elements=interleaverElements
  Matrix Interleaver : commblkintrlv2/Matrix Interleaver  Nrows=interleaverRows  Ncols=interleaverCols
  Rectangular QAM Modulator Baseband : commdigbbndam2/Rectangular QAM Modulator Baseband  M=modOrder  InType=Bit  Enc=Gray  PowType=Average Power  MinDist=2  AvgPow=1  PeakPow=1  Ph=0  numSamp=1
  Zero Pad : dspsigops/Zero Pad  padSigAt=End  zpadAlong=Columns  padNumOutRowsSpecMethod=User-specified  numOutRows=Nb  padNumOutColsSpecMethod=User-specified  numOutCols=1  trunc_flag=None
      settings: AttributesFormatString=\n
  txsig : Outport
  wires:
  Rectangular QAM Modulator Baseband/1 -> Gain1/1
  Gain1/1 -> txsig/1
  txdata/1 -> Zero Pad/1
  Matrix Interleaver/1 -> General Block Interleaver/1
  General Block Interleaver/1 -> Rectangular QAM Modulator Baseband/1
  Zero Pad/1 -> Matrix Interleaver/1

== system ieee80211n/ModulatorBank/ModulatorSS1/Modulator 2 ==
  txdata : Inport  Port=1  LatchInput=off
  Enable : EnablePort
  Gain1 : Gain  SaturateOnIntegerOverflow=on
  General Block Interleaver : commblkintrlv2/General Block Interleaver  elements=interleaverElements
  Matrix Interleaver : commblkintrlv2/Matrix Interleaver  Nrows=interleaverRows  Ncols=interleaverCols
  Rectangular QAM Modulator Baseband : commdigbbndam2/Rectangular QAM Modulator Baseband  M=modOrder  InType=Bit  Enc=Gray  PowType=Average Power  MinDist=2  AvgPow=1  PeakPow=1  Ph=0  numSamp=1
  Zero Pad : dspsigops/Zero Pad  padSigAt=End  zpadAlong=Columns  padNumOutRowsSpecMethod=User-specified  numOutRows=Nb  padNumOutColsSpecMethod=User-specified  numOutCols=1  trunc_flag=None
      settings: AttributesFormatString=\n
  txsig : Outport
  wires:
  Rectangular QAM Modulator Baseband/1 -> Gain1/1
  Gain1/1 -> txsig/1
  txdata/1 -> Zero Pad/1
  Zero Pad/1 -> Matrix Interleaver/1
  Matrix Interleaver/1 -> General Block Interleaver/1
  General Block Interleaver/1 -> Rectangular QAM Modulator Baseband/1

== system ieee80211n/ModulatorBank/ModulatorSS1/Modulator 3 ==
  txdata : Inport  Port=1  LatchInput=off
  Enable : EnablePort
  Gain1 : Gain  SaturateOnIntegerOverflow=on
  General Block Interleaver : commblkintrlv2/General Block Interleaver  elements=interleaverElements
  Matrix Interleaver : commblkintrlv2/Matrix Interleaver  Nrows=interleaverRows  Ncols=interleaverCols
  Rectangular QAM Modulator Baseband : commdigbbndam2/Rectangular QAM Modulator Baseband  M=modOrder  InType=Bit  Enc=Gray  PowType=Average Power  MinDist=2  AvgPow=1  PeakPow=1  Ph=0  numSamp=1
  Zero Pad : dspsigops/Zero Pad  padSigAt=End  zpadAlong=Columns  padNumOutRowsSpecMethod=User-specified  numOutRows=Nb  padNumOutColsSpecMethod=User-specified  numOutCols=1  trunc_flag=None
      settings: AttributesFormatString=\n
  txsig : Outport
  wires:
  Rectangular QAM Modulator Baseband/1 -> Gain1/1
  Gain1/1 -> txsig/1
  txdata/1 -> Zero Pad/1
  Zero Pad/1 -> Matrix Interleaver/1
  Matrix Interleaver/1 -> General Block Interleaver/1
  General Block Interleaver/1 -> Rectangular QAM Modulator Baseband/1

== system ieee80211n/ModulatorBank/ModulatorSS1/Modulator 4 ==
  txdata : Inport  Port=1  LatchInput=off
  Enable : EnablePort
  Gain1 : Gain  SaturateOnIntegerOverflow=on
  General Block Interleaver : commblkintrlv2/General Block Interleaver  elements=interleaverElements
  Matrix Interleaver : commblkintrlv2/Matrix Interleaver  Nrows=interleaverRows  Ncols=interleaverCols
  Rectangular QAM Modulator Baseband : commdigbbndam2/Rectangular QAM Modulator Baseband  M=modOrder  InType=Bit  Enc=Gray  PowType=Average Power  MinDist=2  AvgPow=1  PeakPow=1  Ph=0  numSamp=1
  Zero Pad : dspsigops/Zero Pad  padSigAt=End  zpadAlong=Columns  padNumOutRowsSpecMethod=User-specified  numOutRows=Nb  padNumOutColsSpecMethod=User-specified  numOutCols=1  trunc_flag=None
      settings: AttributesFormatString=\n
  txsig : Outport
  wires:
  Rectangular QAM Modulator Baseband/1 -> Gain1/1
  Gain1/1 -> txsig/1
  txdata/1 -> Zero Pad/1
  Zero Pad/1 -> Matrix Interleaver/1
  Matrix Interleaver/1 -> General Block Interleaver/1
  General Block Interleaver/1 -> Rectangular QAM Modulator Baseband/1

== system ieee80211n/ModulatorBank/ModulatorSS1/Modulator 5 ==
  txdata : Inport  Port=1  LatchInput=off
  Enable : EnablePort
  Gain1 : Gain  SaturateOnIntegerOverflow=on
  General Block Interleaver : commblkintrlv2/General Block Interleaver  elements=interleaverElements
  Matrix Interleaver : commblkintrlv2/Matrix Interleaver  Nrows=interleaverRows  Ncols=interleaverCols
  Rectangular QAM Modulator Baseband : commdigbbndam2/Rectangular QAM Modulator Baseband  M=modOrder  InType=Bit  Enc=Gray  PowType=Average Power  MinDist=2  AvgPow=1  PeakPow=1  Ph=0  numSamp=1
  Zero Pad : dspsigops/Zero Pad  padSigAt=End  zpadAlong=Columns  padNumOutRowsSpecMethod=User-specified  numOutRows=Nb  padNumOutColsSpecMethod=User-specified  numOutCols=1  trunc_flag=None
      settings: AttributesFormatString=\n
  txsig : Outport
  wires:
  Rectangular QAM Modulator Baseband/1 -> Gain1/1
  Gain1/1 -> txsig/1
  txdata/1 -> Zero Pad/1
  Zero Pad/1 -> Matrix Interleaver/1
  Matrix Interleaver/1 -> General Block Interleaver/1
  General Block Interleaver/1 -> Rectangular QAM Modulator Baseband/1
